simulink model "JohnnyDiagram"  (R2023a)
settings: Solver=VariableStepAuto  StartTime=0.0  StopTime=10.0  RelTol=1e-3
libraries: simulink x7
settings Model: Creator=TELEPUZ  LastModifiedBy=TELEPUZ

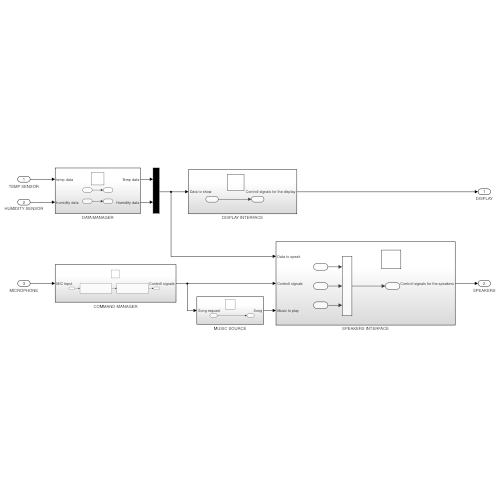
[thumbnail: Simulink's stored preview of the top-level diagram]
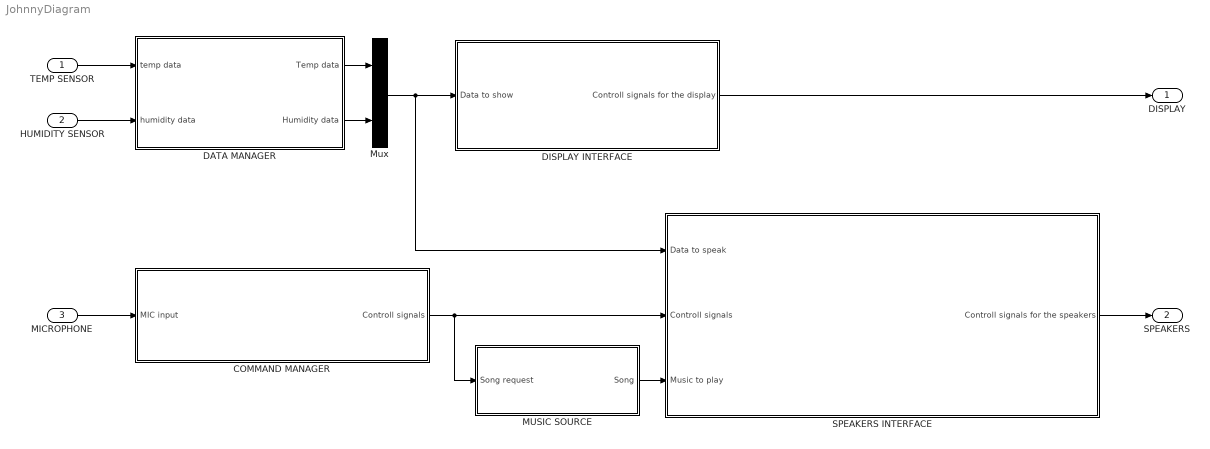
== system JohnnyDiagram ==
  TEMP SENSOR : Inport
  HUMIDITY SENSOR : Inport  Port=2
  MICROPHONE : Inport  Port=3
  COMMAND MANAGER : Subsystem
  DATA MANAGER : Subsystem
  DISPLAY INTERFACE : Subsystem
  MUSIC SOURCE : Subsystem
  Mux : Mux  Inputs=2
  SPEAKERS INTERFACE : Subsystem
  DISPLAY : Outport
  SPEAKERS : Outport  Port=2
  wires:
  TEMP SENSOR/1 -> DATA MANAGER/1(temp data)
  HUMIDITY SENSOR/1 -> DATA MANAGER/2(humidity data)
  MICROPHONE/1 -> COMMAND MANAGER/1(MIC input)
  DATA MANAGER/1(Temp data) -> Mux/1
  DATA MANAGER/2(Humidity data) -> Mux/2
  Mux/1 -> DISPLAY INTERFACE/1(Data to show), SPEAKERS INTERFACE/1(Data to speak)
  DISPLAY INTERFACE/1(Controll signals for the display) -> DISPLAY/1
  COMMAND MANAGER/1(Controll signals) -> SPEAKERS INTERFACE/2("Controll signals "), MUSIC SOURCE/1(Song request)
  MUSIC SOURCE/1(Song) -> SPEAKERS INTERFACE/3(Music to play)
  SPEAKERS INTERFACE/1(Controll signals for the speakers) -> SPEAKERS/1

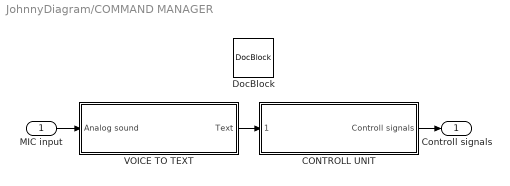
== system JohnnyDiagram/COMMAND MANAGER ==
  MIC input : Inport
  CONTROLL UNIT : Subsystem
  DocBlock : simulink/Model-Wide Utilities/DocBlock  DocumentType=Text
      content=|
      | This block converts analog input to consiquence of words and trying to detect start word there.
      | If it is detected, following consequence of words considers as the command, based on the context of which controll signals for out periphery are formed.
  VOICE TO TEXT : Subsystem
  Controll signals : Outport
  wires:
  MIC input/1 -> VOICE TO TEXT/1(Analog sound)
  VOICE TO TEXT/1(Text) -> CONTROLL UNIT/1(" ")
  CONTROLL UNIT/1(Controll signals) -> Controll signals/1

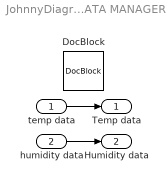
== system JohnnyDiagram/DATA MANAGER ==
  temp data : Inport
  humidity data : Inport  Port=2
  DocBlock : simulink/Model-Wide Utilities/DocBlock  DocumentType=Text
      content=|
      | Data manager gathers and stores measurments from sensors for further using.
  Temp data : Outport
  Humidity data : Outport  Port=2
  wires:
  temp data/1 -> Temp data/1
  humidity data/1 -> Humidity data/1

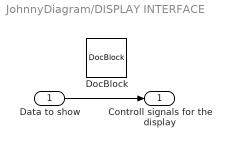
== system JohnnyDiagram/DISPLAY INTERFACE ==
  Data to show : Inport
  DocBlock : simulink/Model-Wide Utilities/DocBlock  DocumentType=Text
      content=|
      | Realizes displaying current humidity, temp, time on the display.
  Controll signals for the display : Outport
  wires:
  Data to show/1 -> Controll signals for the display/1

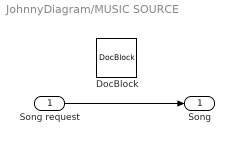
== system JohnnyDiagram/MUSIC SOURCE ==
  Song request : Inport
  DocBlock : simulink/Model-Wide Utilities/DocBlock  DocumentType=Text
      content=|
      | There are two options of the getting music for playing:
      | 1. Store some amount locally, just downloaded from the internet.
      | 2. Spotify request each time for each song.
      |
      | Specific realization is on the team member, who will realize this block.
  Song : Outport
  wires:
  Song request/1 -> Song/1

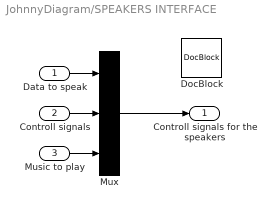
== system JohnnyDiagram/SPEAKERS INTERFACE ==
  Data to speak : Inport
  "Controll signals " : Inport  Port=2
  Music to play : Inport  Port=3
  DocBlock : simulink/Model-Wide Utilities/DocBlock  DocumentType=Text
      content=|
      | Realizes playing of asked info by the User or playing of the music.
  Mux : Mux  Inputs=3
  Controll signals for the speakers : Outport
  wires:
  Data to speak/1 -> Mux/1
  "Controll signals "/1 -> Mux/2
  Music to play/1 -> Mux/3
  Mux/1 -> Controll signals for the speakers/1

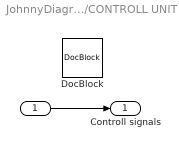
== system JohnnyDiagram/COMMAND MANAGER/CONTROLL UNIT ==
  " " : Inport
  DocBlock : simulink/Model-Wide Utilities/DocBlock  DocumentType=Text
      content=|
      | If start word recognized, following sequence of words considers as a command from the User. Based on which we decide, which output is required.
  Controll signals : Outport
  wires:
  " "/1 -> Controll signals/1

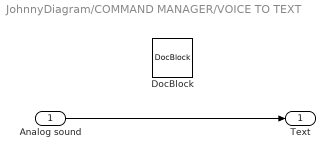
== system JohnnyDiagram/COMMAND MANAGER/VOICE TO TEXT ==
  Analog sound : Inport
  DocBlock : simulink/Model-Wide Utilities/DocBlock  DocumentType=Text
      content=|
      | Converts analog input from the MIC into the text.
  Text : Outport
  wires:
  Analog sound/1 -> Text/1
